simulink model "sys_model"  (R2021a)
settings: Solver=FixedStepDiscrete  StartTime=0.0  StopTime=200  RelTol=1e-3
settings Model: Creator=Rasika Shejul  LastModifiedBy=Rushikesh
settings SolverCC: AlgebraicLoopSolver=TrustRegion
settings DebuggingCC: SFMachineParentedDataDiag=warning

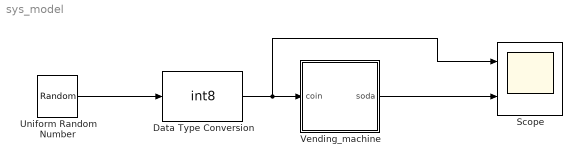
== system sys_model ==
  Data Type Conversion : DataTypeConversion  OutDataTypeStr=int8  RndMeth=Nearest  SaturateOnIntegerOverflow=on
  Scope : Scope  NumInputPorts=2
  Uniform Random Number : UniformRandomNumber  Minimum=0  Maximum=2  Seed=337  SampleTime=10
  Vending_machine : Stateflow chart  TreatAsAtomicUnit=on
  wires:
  Uniform Random Number/1 -> Data Type Conversion/1
  Data Type Conversion/1 -> Vending_machine/1(coin), Scope/1
  Vending_machine/1(soda) -> Scope/2

== stateflow chart sys_model/Vending_machine ==
  settings: stateMachineType=MEALY_MACHINE  initializeOutput=1
  state got_0
  state got_Nickel
  state got_dime
  (default) -> got_0
  got_0 -> got_Nickel [order 1] : [coin==1]{soda=0}
  got_Nickel -> got_0 [order 2] : [coin==2]{soda=1}
  got_0 -> got_dime [order 2] : [coin==2]{soda=0}
  got_dime -> got_0 [order 1] : [coin==1]{soda=1}
  got_Nickel -> got_dime [order 1] : [coin==1]{soda=0}
  got_dime -> got_Nickel [order 2] : [coin==2]{soda=1}
  data: soda output double; coin input int8
